simulink model "controller"  (R2025a)
settings: Solver=FixedStepAuto  StartTime=0.0  StopTime=inf  RelTol=1e-3  EnableMultiTasking=on
libraries: stm32f4xxblockslib x3, stm32blockslib x3, stm32g4xxblockslib x1
settings Model: STM32="{\"AnalogInput\":[{\"ID\":\"controller:164\"},{\"ID\":\"controller:165\"}],\"AnalogOutput\":{\"ID\":\"controller:188\"},\"HardwareInterrupt\":{\"ID\":\"controller:206\"},\"PWMOutput\":{\"ID\":\"controller:214\"},\"UARTRead\":{\"ID\":\"controller:236\"},\"UARTWrite\":{\"ID\":\"controller:237\"}}"  Creator=GNKRISHNAN  LastModifiedBy=GNKRISHNAN
settings SolverCC: AutoInsertRateTranBlk=on
settings OptimizationCC: DefaultParameterBehavior=Inlined  EnhancedBackFolding=on  PassReuseOutputArgsAs=Individual arguments  ZeroExternalMemoryAtStartup=off  ZeroInternalMemoryAtStartup=off  MaxStackSize=512  OptimizeBlockOrder=speed  DifferentSizesBufferReuse=on  OptimizationCustomize=off  EfficientTunableParamExpr=on
settings DebuggingCC: ParameterTunabilityLossMsg=error
settings HardwareCC: ProdBitPerPointer=32.0  ProdBitPerSizeT=32.0  ProdBitPerPtrDiffT=32.0  ProdLargestAtomicInteger=Long  ProdLargestAtomicFloat=Double  ProdWordSize=32.0  ProdLongLongMode=on  ProdHWDeviceType=ARM Compatible->ARM Cortex-M
settings SFSimCC: MATLABDynamicMemAlloc=off
settings RTWCC: SystemTargetFile=ert.tlc  HardwareBoard=STM32G4xx Based  TemplateMakefile=ert_default_tmf  CustomHeaderCode="#include \"stm32g4xx_ll_usart.h\""  CustomInclude=C:\Users\GNKRISHNAN\STM32Cube\Repository\STM32Cube_FW_G4_V1.6.0\Drivers\STM32G4xx_HAL_Driver\Inc  Toolchain=GNU Tools for ARM Embedded Processors  Description=Embedded Coder
settings CodeAppCC: ForceParamTrailComments=on  IgnoreCustomStorageClasses=off  OperatorAnnotations=on  SimulinkDataObjDesc=on  SFDataObjDesc=on  InsertBlockDesc=on
settings ERTTargetCC: ExtModeTransport=3.0  ExtModeStaticAllocSize=2048.0  TargetLangStandard=C99 (ISO)  CodeReplacementLibrary=ARM Cortex-M

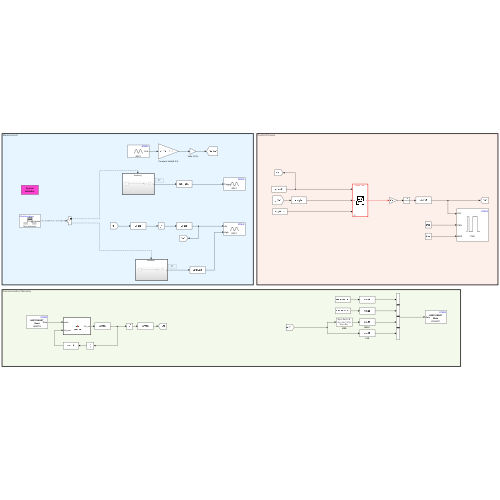
[thumbnail: Simulink's stored preview of the top-level diagram]
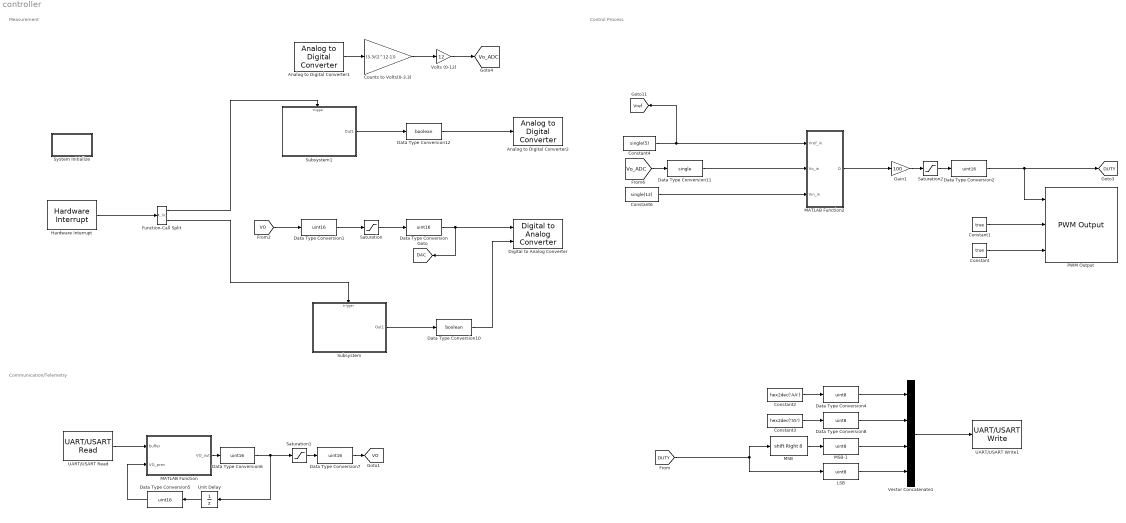
== system controller ==
  note: Control Process
  note: Measurement
  note: Communication/Telemetry
  Analog to Digital Converter1 : stm32f4xxblockslib/Analog to Digital Converter  ADCModule=ADC1  ConversionGroup=Regular  TriggerMode=Read results only  NumberOfConversions=1  EnableBufferConv=off  BufferLength=1  OutputStatus=off  SampleTime=-1  EnableSimPort=off  hoistedMaskSrc=ECSoC/ECSimCodegen/Analog to Digital Converter
  Analog to Digital Converter2 : stm32f4xxblockslib/Analog to Digital Converter  ADCModule=ADC1  ConversionGroup=Regular  TriggerMode=Trigger only  NumberOfConversions=1  EnableBufferConv=off  BufferLength=1  OutputStatus=off  SampleTime=-1  EnableSimPort=off  hoistedMaskSrc=ECSoC/ECSimCodegen/Analog to Digital Converter
  Constant : Constant  Value=true
  Constant1 : Constant  Value=true
  Constant2 : Constant  Value=hex2dec('AA')
  Constant3 : Constant  Value=hex2dec('55')
  Constant4 : Constant  Value=single(5)
  Constant6 : Constant  Value=single(12)
  Counts to Volts(0-3.3) : Gain  Gain=(3.3/(2^12-1))  ParamDataTypeStr=single
  Data Type Conversion{,1..2,5..7} (6 alike) : DataTypeConversion  OutDataTypeStr=uint16  SaturateOnIntegerOverflow=off  RndMeth=Floor
  Data Type Conversion10 : DataTypeConversion  OutDataTypeStr=boolean  SaturateOnIntegerOverflow=off  RndMeth=Floor
  Data Type Conversion11 : DataTypeConversion  OutDataTypeStr=single  SaturateOnIntegerOverflow=off  RndMeth=Floor
  Data Type Conversion12 : DataTypeConversion  OutDataTypeStr=boolean  SaturateOnIntegerOverflow=off  RndMeth=Floor
  Data Type Conversion4 : DataTypeConversion  OutDataTypeStr=uint8  SaturateOnIntegerOverflow=off  RndMeth=Floor
  Data Type Conversion8 : DataTypeConversion  OutDataTypeStr=uint8  SaturateOnIntegerOverflow=off  RndMeth=Floor
  Digital to Analog Converter : stm32blockslib/Digital to Analog Converter  DACModule=DAC1  TriggerType=Write and trigger  ChannelGroup=Channel1  waveGenEnable=off  waveType=Noise/Triangular  TriggerEnable=on  stepTriggerEnable=on  resetTriggerEnable=on  TrigConfig=Independent trigger  DataLength=12 bits  DataAlignment=Right alignment  dacEnable=off  OutputStatus=off
      settings: LibrarySourceBlock=stm32g4xxblockslib/Digital to Analog Converter
  Function-Call Split : FunctionCallSplit  IconShape=distinctive  NumOutputPorts=2  OutputPortLayout=default
  Gain1 : Gain  Gain=100
  Hardware Interrupt : stm32g4xxblockslib/Hardware Interrupt  ISRGroup=Timer (TIM)  ISRName=TIM3_IRQHandler  ISRNumber=44  EventsList={ 'on', 'TIM3 Update', '1'; 'off', 'TIM3 CC1', '2'; 'off', 'TIM3 CC2', '3'; 'off', 'TIM3 CC3', '4'; 'off', 'TIM3 CC4', '5'; 'off', 'TIM3 Trigger', '6'; 'off', 'TIM3 DIR', '7'; 'off', 'TIM3 IDX', '8'; 'off', 'TIM3 IERR', '9'; 'off', 'TIM3 TERR', '10'; 'off', 'Custom event', '11' }  SelectedEvents={'TIM3 Update'}  TaskPriority=30  DisablePreemption=off  ClearInterruptFlagsAtEndOfEvent=off  InterruptDefinitionFile=$(TARGET_ROOT)/registry/interrupts/STM32F4xxBased_interrupts.xml  HardwareBoard=STM32G4xx Based  EnableSimPort=off
  LSB : DataTypeConversion  OutDataTypeStr=uint8  SaturateOnIntegerOverflow=off  RndMeth=Floor
  MATLAB Function : MATLAB Function  TreatAsAtomicUnit=on
  MATLAB Function2 : MATLAB Function  TreatAsAtomicUnit=on
  MSB : ArithShift  BitShiftNumber=8  BitShiftDirection=Right
  MSB-1 : DataTypeConversion  OutDataTypeStr=uint8  SaturateOnIntegerOverflow=off  RndMeth=Floor
  PWM Output : stm32f4xxblockslib/PWM Output  ProcessorFamily=STM32G4  TimerModule=TIM1  DutycycleUnits=Percentage  EnableChannel1=on  EnableCaptureCompare1Input=off  EnableCaptureCompare1ComplementaryInput=off  EnableOutputCompare1ModeInput=off  EnableChannel2=off  EnableCaptureCompare2Input=off  EnableCaptureCompare2ComplementaryInput=off  EnableOutputCompare2ModeInput=off  EnableChannel3=off  EnableCaptureCompare3Input=off  EnableCaptureCompare3ComplementaryInput=off  EnableOutputCompare3ModeInput=off  EnableChannel4=off  EnableCaptureCompare4Input=off  EnableCaptureCompare4ComplementaryInput=off  EnableOutputCompare4ModeInput=off  EnableChannel5=off  EnableCaptureCompare5Input=off  EnableOutputCompare5ModeInput=off  EnableChannel6=off  EnableCaptureCompare6Input=off  EnableOutputCompare6ModeInput=off  EnableCounterInput=on  EnableMainOutputInput=on  EnableFrequencyInput=off  SetRCAfterCE=off  OutputDirection=off  OutputMainOutputEnableStatus=off  SampleTime=0.1  EnableSimPort=off  EnableUpdateEvent=off  EnableCaptureCompare1Event=off  EnableCaptureCompare2Event=off  EnableCaptureCompare3Event=off  EnableCaptureCompare4Event=off  EnableTriggerEvent=off  EnableBreakEvent=off  EnableBreakEvent2=off  hoistedMaskSrc=ECSoC/ECSimCodegen/PWM Output
      settings: LibrarySourceBlock=stm32g4xxblockslib/PWM Output
  Saturation : Saturate  UpperLimit=4095  LowerLimit=0
  Saturation1 : Saturate  UpperLimit=4095  LowerLimit=0
  Saturation2 : Saturate  UpperLimit=100  LowerLimit=0
  Subsystem : Subsystem
  Subsystem1 : Subsystem
  System Initialize : Subsystem  mask(System Initialize){ShowInLibBrowser=0}
      mask prompts: ShowInLibBrowser "Simulink:masks:CustCodeMaskParam1_MP"
      settings: CopyFcn=cccopyfcn(gcb)  OpenFcn=ccopenfcn('System Initialize Function')
      mask Help: eval('feval(''rtwprivate'',''rtwhelpview'',''rtw_sys_initialize_block'')');
      mask Display: disp('System\nInitialize');
  UART/USART Read : stm32blockslib/UART//USART Read  UARTModule=USART3  DataType=uint8  DataLength=10  BlockingMode=off  BlockingTimeout=0.1  OutputLength=off  OutputStatus=off  SampleTime=-1
      settings: LibrarySourceBlock=stm32g4xxblockslib/UART//USART Read
  UART/USART Write1 : stm32blockslib/UART//USART Write  UARTModule=LPUART1  LengthOfDataToSend=off  BlockingMode=off  BlockingTimeout=100e-3  OutputStatus=off
      settings: LibrarySourceBlock=stm32g4xxblockslib/UART//USART Write
  Unit Delay : UnitDelay  InitialCondition=uint16(0)  SampleTime=-1  HasFrameUpgradeWarning=on
  Vector Concatenate1 : Concatenate  NumInputs=4
  Volts (0-12) : Gain  Gain=12
  tag scope: DAC=global, DUTY=global, VO=global, Vo_ADC=global, Vref=global
  wires:
  Data Type Conversion2/1 -> [DUTY], PWM Output/1
  Unit Delay/1 -> Data Type Conversion5/1
  Data Type Conversion1/1 -> Saturation/1
  Data Type Conversion12/1 -> Analog to Digital Converter2/1
  Vector Concatenate1/1 -> UART/USART Write1/1
  Hardware Interrupt/1 -> Function-Call Split/1
  Data Type Conversion10/1 -> Digital to Analog Converter/2
  Data Type Conversion4/1 -> Vector Concatenate1/1
  Data Type Conversion8/1 -> Vector Concatenate1/2
  [Vo_ADC] -> Data Type Conversion11/1
  LSB/1 -> Vector Concatenate1/4
  MATLAB Function2/1(D) -> Gain1/1
  Saturation1/1 -> Data Type Conversion7/1
  Data Type Conversion6/1 -> Saturation1/1, Unit Delay/1
  MSB-1/1 -> Vector Concatenate1/3
  [VO] -> Data Type Conversion1/1
  Analog to Digital Converter1/1 -> Counts to Volts(0-3.3)/1
  Data Type Conversion7/1 -> [VO]
  Data Type Conversion5/1 -> MATLAB Function/2(VO_prev)
  UART/USART Read/1 -> MATLAB Function/1(buffer)
  Constant2/1 -> Data Type Conversion4/1
  Data Type Conversion/1 -> Digital to Analog Converter/1, [DAC]
  Saturation/1 -> Data Type Conversion/1
  Gain1/1 -> Saturation2/1
  [DUTY] -> MSB/1, LSB/1
  MSB/1 -> MSB-1/1
  Counts to Volts(0-3.3)/1 -> Volts (0-12)/1
  Constant/1 -> PWM Output/3
  Function-Call Split/2 -> Subsystem/Trigger
  Constant3/1 -> Data Type Conversion8/1
  Function-Call Split/1 -> Subsystem1/Trigger
  Volts (0-12)/1 -> [Vo_ADC]
  Subsystem1/1(Out1) -> Data Type Conversion12/1
  MATLAB Function/1(VO_out) -> Data Type Conversion6/1
  Constant6/1 -> MATLAB Function2/3(Vin_in)
  Data Type Conversion11/1 -> MATLAB Function2/2(Vo_in)
  Constant1/1 -> PWM Output/2
  Saturation2/1 -> Data Type Conversion2/1
  Constant4/1 -> MATLAB Function2/1(Vref_in), [Vref]
  Subsystem/1(Out1) -> Data Type Conversion10/1

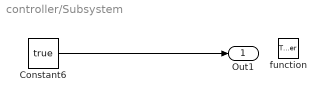
== system controller/Subsystem ==
  function : TriggerPort  TriggerType=function-call  VariantControl=(inherit)
  Constant6 : Constant  Value=true
  Out1 : Outport
  wires:
  Constant6/1 -> Out1/1

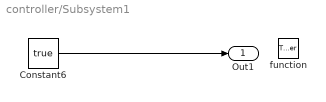
== system controller/Subsystem1 ==
  function : TriggerPort  TriggerType=function-call  VariantControl=(inherit)
  Constant6 : Constant  Value=true
  Out1 : Outport
  wires:
  Constant6/1 -> Out1/1

== system controller/System Initialize ==

== matlab function controller/MATLAB Function ==
  data: buffer input; VO_out output; VO_prev input
function VO_out = parse_rx(buffer, VO_prev)
    % EXPLICIT CAST: Forces VO_out to be a 16-bit integer in C-code
    VO_out = uint16(VO_prev); 
    
    len = length(buffer);
    
    for i = 1:(len - 3)
        if buffer(i) == 170 && buffer(i+1) == 86
            MSB = uint16(buffer(i+2));
            LSB = uint16(buffer(i+3));
            
            % bitor also outputs a uint16, so the memory types now match perfectly
            VO_out = bitor(bitshift(MSB, 8), LSB);
            break; 
        end
    end
end

== matlab function controller/MATLAB Function2 ==
  data: Vref_in input; D output; Vo_in input; Vin_in input
function D = buck_controller(Vref_in, Vo_in, Vin_in)
%#codegen
% Feedforward + PI with Sanity Shield & Directional Anti-Windup
% Plant: fs = 20kHz | UART Co-Simulation Safe

persistent int_v
persistent D_prev
persistent Vo_prev
persistent is_initialized

%% -------- Constants --------
Kp        = single(0.005);
Ki_step   = single(1e-5); 
Dmax      = single(0.95);
Dmin      = single(0.00);

% Hysteresis Parameters
Vband     = single(0.30);   % +/- 0.3V deadband for Proportional Gain
D_hyst    = single(0.002);  % Output filter threshold

%% -------- Initialization --------
if isempty(is_initialized)
    D_prev         = single(Vref_in / Vin_in); % Start at feedforward
    int_v          = single(0.0);
    Vo_prev        = single(0.0);
    is_initialized = true;
end

%% -------- Type Casting & Sanity Shield --------
Vref   = single(Vref_in);
Vin    = single(Vin_in);
Vo_raw = single(Vo_in);

% OUTLIER REJECTION: Reject corrupted UART packets.
% A buck converter cannot realistically output more than 1.5x Vin during a transient,
% nor can it output negative voltage. Anything outside this is a dropped-byte error.
if Vo_raw > (Vin * 1.5) || Vo_raw < 0.0
    Vo = Vo_prev; % Ignore garbage, use last known good value
else
    Vo = Vo_raw;
    Vo_prev = Vo;
end

%% -------- Feedforward & Error --------
D_ff = Vref / Vin;
ev   = Vref - Vo;

% Hard limit the error to prevent any minor slips from winding the integrator
if ev > Vref
    ev = Vref;
elseif ev < -Vref
    ev = -Vref;
end

%% -------- Gain Scheduling --------
if abs(ev) < Vband
    Kp_active = single(0.0);
else
    Kp_active = Kp;
end

%% -------- PI Correction --------
D_unclamped = D_ff + (Kp_active * ev) + int_v;

%% -------- Directional Anti-Windup --------
% Only allow integration if it pulls the system AWAY from the saturation wall
if D_unclamped > Dmax
    D_ideal = Dmax;
    if ev < 0.0
        int_v = int_v + (ev * Ki_step);
    end
elseif D_unclamped < Dmin
    D_ideal = Dmin;
    if ev > 0.0
        int_v = int_v + (ev * Ki_step);
    end
else
    D_ideal = D_unclamped;
    int_v = int_v + (ev * Ki_step);
end

%% -------- Duty Change Threshold --------
if abs(D_ideal - D_prev) < D_hyst
    D = D_prev;
else
    D = D_ideal;
    D_prev = D;
end

end
